simulink model "outerControllerTuning"  (R2018a)
settings: Solver=ode15s  StartTime=0.0  StopTime=t  RelTol=1e-3
values from neighbouring files (symbols this model uses):
  d = 2.4*10^-3    (= 0.0024)    [innerInit.m]    (also in outerInit.m)
  g = 9.81    [innerInit.m]    (also in outerInit.m)
  Ixx = 5.9*10^-3    (= 0.0059)    [innerInit.m]    (also in outerInit.m)
  Iyy = 5.9*10^-3    (= 0.0059)    [innerInit.m]    (also in outerInit.m)
  Izz = 1.16*10^-3    (= 0.00116)    [innerInit.m]    (also in outerInit.m)
  kr = 0.1    [innerInit.m]    (also in outerInit.m)
  kt = 0.1    [innerInit.m]    (also in outerInit.m)
  l = 0.255    [innerInit.m]    (also in outerInit.m)
  m = 0.5    [innerInit.m]    (also in outerInit.m)
  x0 = 1    [innerInit.m]    (also in outerInit.m = 2)
  x_coeff = A^-1*x_constr    [outerInit.m]
  xd = 0    [innerInit.m]    (also in outerInit.m)
  xdot0 = 0    [outerInit.m]
  y0 = 1    [innerInit.m]    (also in outerInit.m = 3)
  y_coeff = A^-1*y_constr    [outerInit.m]
  yd = 0    [innerInit.m]    (also in outerInit.m)
  ydot0 = 0    [outerInit.m]
  z0 = 0    [innerInit.m]    (also in outerInit.m = 4)
  z_coeff = A^-1*z_constr    [outerInit.m]
  zd = 10    [innerInit.m]    (also in outerInit.m = 0)
  zdot0 = 0    [outerInit.m]
libraries: simulink x4
settings Model: Creator=dinies33  LastModifiedBy=giuseppe

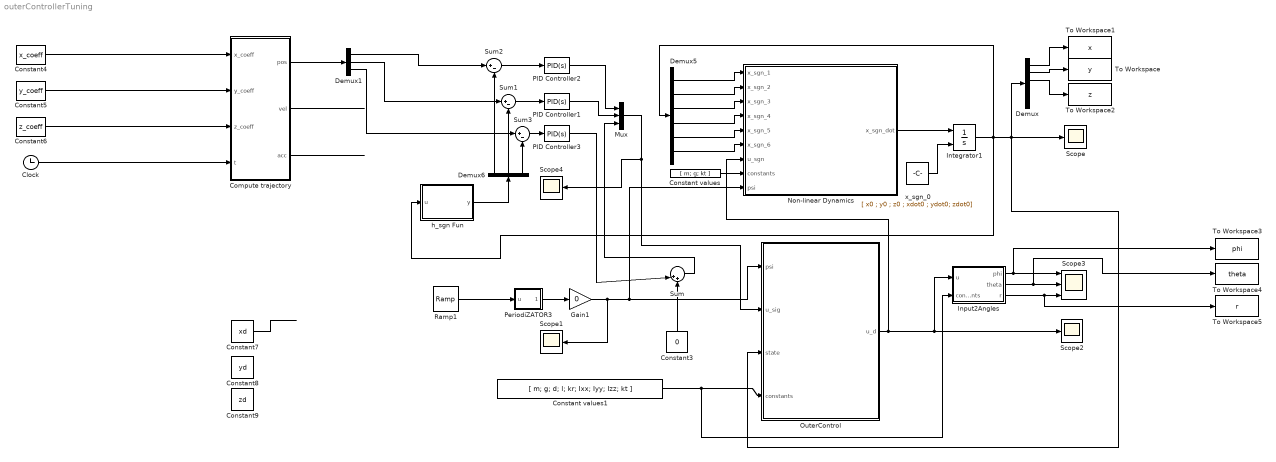
== system outerControllerTuning ==
  Clock : Clock
  Compute trajectory : MATLAB Function  TreatAsAtomicUnit=on
  Constant values : Constant  Value=[ m; g; kt ]
  Constant values1 : Constant  Value=[ m; g; d; l; kr; Ixx; Iyy; Izz; kt ]
  Constant3 : Constant  Value=0
  Constant4 : Constant  Value=x_coeff
  Constant5 : Constant  Value=y_coeff
  Constant6 : Constant  Value=z_coeff
  Constant7 : Constant  Value=xd
  Constant8 : Constant  Value=yd
  Constant9 : Constant  Value=zd
  Demux : Demux  Outputs=6
  Demux1 : Demux  Outputs=3
  Demux5 : Demux  Outputs=6
  Demux6 : Demux  Outputs=3
  Gain1 : Gain  Gain=0
  Input2Angles : MATLAB Function  TreatAsAtomicUnit=on
  Integrator1 : Integrator  InitialConditionSource=external
  Mux : Mux  Inputs=3
  Non-linear Dynamics : MATLAB Function  TreatAsAtomicUnit=on
  OuterControl : MATLAB Function  TreatAsAtomicUnit=on
  PID Controller1 : simulink/Continuous/PID Controller  Controller=PID  TimeDomain=Continuous-time  SampleTime=-1  IntegratorMethod=Forward Euler  FilterMethod=Forward Euler  Form=Parallel  UseFilter=on  ControllerParametersSource=internal  P=0.942155734377191  I=0.0299673249963071  D=20  N=509.539625142761  InitialConditionSource=internal  InitialConditionForIntegrator=0  InitialConditionForFilter=0  ExternalReset=none  LimitOutput=off  UpperSaturationLimit=inf  LowerSaturationLimit=-inf  LinearizeAsGain=on  AntiWindupMode=none  Kb=1  TrackingMode=off  Kt=1  PParamMin=[]  PParamMax=[]  IParamMin=[]  IParamMax=[]  DParamMin=[]  DParamMax=[]  NParamMin=[]  NParamMax=[]  KbParamMin=[]  KbParamMax=[]  KtParamMin=[]  KtParamMax=[]  POutMin=[]  POutMax=[]  IOutMin=[]  IOutMax=[]  DOutMin=[]  DOutMax=[]  NOutMin=[]  NOutMax=[]  KbOutMin=[]  KbOutMax=[]  KtOutMin=[]  KtOutMax=[]  IntegratorOutMin=[]  IntegratorOutMax=[]  FilterOutMin=[]  FilterOutMax=[]  SumOutMin=[]  SumOutMax=[]  SumI1OutMin=[]  SumI1OutMax=[]  SumI2OutMin=[]  SumI2OutMax=[]  SumI3OutMin=[]  SumI3OutMax=[]  SumDOutMin=[]  SumDOutMax=[]  SaturationOutMin=[]  SaturationOutMax=[]  IntegratorContinuousStateAttributes=''  IntegratorStateMustResolveToSignalObject=off  IntegratorRTWStateStorageClass=Auto  FilterContinuousStateAttributes=''  FilterStateMustResolveToSignalObject=off  FilterRTWStateStorageClass=Auto  DifferentiatorICPrevScaledInput=0  DifferentiatorOutMin=[]  DifferentiatorOutMax=[]  FilterDiffOutCoefMin=[]  FilterDiffOutCoefMax=[]  SumDenOutMin=[]  SumDenOutMax=[]  SumNumOutMin=[]  SumNumOutMax=[]  ReciprocalOutMin=[]  ReciprocalOutMax=[]  DivideOutMin=[]  DivideOutMax=[]  TunerSelectOption=Transfer Function Based (PID Tuner App)
  PID Controller2 : simulink/Continuous/PID Controller  Controller=PID  TimeDomain=Continuous-time  SampleTime=-1  IntegratorMethod=Forward Euler  FilterMethod=Forward Euler  Form=Parallel  UseFilter=on  ControllerParametersSource=internal  P=0.942155734377191  I=0.0299673249963071  D=20  N=509.539625142761  InitialConditionSource=internal  InitialConditionForIntegrator=0  InitialConditionForFilter=0  ExternalReset=none  LimitOutput=off  UpperSaturationLimit=inf  LowerSaturationLimit=-inf  LinearizeAsGain=on  AntiWindupMode=none  Kb=1  TrackingMode=off  Kt=1  PParamMin=[]  PParamMax=[]  IParamMin=[]  IParamMax=[]  DParamMin=[]  DParamMax=[]  NParamMin=[]  NParamMax=[]  KbParamMin=[]  KbParamMax=[]  KtParamMin=[]  KtParamMax=[]  POutMin=[]  POutMax=[]  IOutMin=[]  IOutMax=[]  DOutMin=[]  DOutMax=[]  NOutMin=[]  NOutMax=[]  KbOutMin=[]  KbOutMax=[]  KtOutMin=[]  KtOutMax=[]  IntegratorOutMin=[]  IntegratorOutMax=[]  FilterOutMin=[]  FilterOutMax=[]  SumOutMin=[]  SumOutMax=[]  SumI1OutMin=[]  SumI1OutMax=[]  SumI2OutMin=[]  SumI2OutMax=[]  SumI3OutMin=[]  SumI3OutMax=[]  SumDOutMin=[]  SumDOutMax=[]  SaturationOutMin=[]  SaturationOutMax=[]  IntegratorContinuousStateAttributes=''  IntegratorStateMustResolveToSignalObject=off  IntegratorRTWStateStorageClass=Auto  FilterContinuousStateAttributes=''  FilterStateMustResolveToSignalObject=off  FilterRTWStateStorageClass=Auto  DifferentiatorICPrevScaledInput=0  DifferentiatorOutMin=[]  DifferentiatorOutMax=[]  FilterDiffOutCoefMin=[]  FilterDiffOutCoefMax=[]  SumDenOutMin=[]  SumDenOutMax=[]  SumNumOutMin=[]  SumNumOutMax=[]  ReciprocalOutMin=[]  ReciprocalOutMax=[]  DivideOutMin=[]  DivideOutMax=[]  TunerSelectOption=Transfer Function Based (PID Tuner App)
  PID Controller3 : simulink/Continuous/PID Controller  Controller=PID  TimeDomain=Continuous-time  SampleTime=-1  IntegratorMethod=Forward Euler  FilterMethod=Forward Euler  Form=Parallel  UseFilter=on  ControllerParametersSource=internal  P=0.942155734377191  I=0.0299673249963071  D=30  N=509.539625142761  InitialConditionSource=internal  InitialConditionForIntegrator=0  InitialConditionForFilter=0  ExternalReset=none  LimitOutput=off  UpperSaturationLimit=inf  LowerSaturationLimit=-inf  LinearizeAsGain=on  AntiWindupMode=none  Kb=1  TrackingMode=off  Kt=1  PParamMin=[]  PParamMax=[]  IParamMin=[]  IParamMax=[]  DParamMin=[]  DParamMax=[]  NParamMin=[]  NParamMax=[]  KbParamMin=[]  KbParamMax=[]  KtParamMin=[]  KtParamMax=[]  POutMin=[]  POutMax=[]  IOutMin=[]  IOutMax=[]  DOutMin=[]  DOutMax=[]  NOutMin=[]  NOutMax=[]  KbOutMin=[]  KbOutMax=[]  KtOutMin=[]  KtOutMax=[]  IntegratorOutMin=[]  IntegratorOutMax=[]  FilterOutMin=[]  FilterOutMax=[]  SumOutMin=[]  SumOutMax=[]  SumI1OutMin=[]  SumI1OutMax=[]  SumI2OutMin=[]  SumI2OutMax=[]  SumI3OutMin=[]  SumI3OutMax=[]  SumDOutMin=[]  SumDOutMax=[]  SaturationOutMin=[]  SaturationOutMax=[]  IntegratorContinuousStateAttributes=''  IntegratorStateMustResolveToSignalObject=off  IntegratorRTWStateStorageClass=Auto  FilterContinuousStateAttributes=''  FilterStateMustResolveToSignalObject=off  FilterRTWStateStorageClass=Auto  DifferentiatorICPrevScaledInput=0  DifferentiatorOutMin=[]  DifferentiatorOutMax=[]  FilterDiffOutCoefMin=[]  FilterDiffOutCoefMax=[]  SumDenOutMin=[]  SumDenOutMax=[]  SumNumOutMin=[]  SumNumOutMax=[]  ReciprocalOutMin=[]  ReciprocalOutMax=[]  DivideOutMin=[]  DivideOutMax=[]  TunerSelectOption=Transfer Function Based (PID Tuner App)
  PeriodiZATOR3 : MATLAB Function  TreatAsAtomicUnit=on
  Ramp1 : simulink/Sources/Ramp  slope=0.3  start=0  InitialOutput=0
  Scope{,1..2,4} (4 alike) : Scope
  Scope3 : Scope  NumInputPorts=3
  Sum : Sum  Inputs=||++
  Sum1 : Sum  Inputs=|+-
  Sum2 : Sum  Inputs=|+-
  Sum3 : Sum  Inputs=|+-
  To Workspace : ToWorkspace  VariableName=y  SaveFormat=Timeseries  SampleTime=-1
  To Workspace1 : ToWorkspace  VariableName=x  SaveFormat=Timeseries  SampleTime=-1
  To Workspace2 : ToWorkspace  VariableName=z  SaveFormat=Timeseries  SampleTime=-1
  To Workspace3 : ToWorkspace  VariableName=phi  SaveFormat=Timeseries  SampleTime=-1
  To Workspace4 : ToWorkspace  VariableName=theta  SaveFormat=Timeseries  SampleTime=-1
  To Workspace5 : ToWorkspace  VariableName=r  SaveFormat=Timeseries  SampleTime=-1
  h_sgn Fun : MATLAB Function  TreatAsAtomicUnit=on
  x_sgn_0 : Constant  Value=[ x0 ; y0 ; z0 ; xdot0 ; ydot0; zdot0]
  wires:
  Constant values/1 -> Non-linear Dynamics/8(constants)
  Non-linear Dynamics/1(x_sgn_dot) -> Integrator1/1
  Integrator1/1 -> Demux5/1, OuterControl/3(state), Demux/1, Scope/1, h_sgn Fun/1(u)
  x_sgn_0/1 -> Integrator1/2
  Demux5/1 -> Non-linear Dynamics/1(x_sgn_1)
  Demux5/2 -> Non-linear Dynamics/2(x_sgn_2)
  Demux5/3 -> Non-linear Dynamics/3(x_sgn_3)
  Demux5/4 -> Non-linear Dynamics/4(x_sgn_4)
  Demux5/5 -> Non-linear Dynamics/5(x_sgn_5)
  Demux5/6 -> Non-linear Dynamics/6(x_sgn_6)
  Demux6/1 -> Sum2/2
  Demux6/2 -> Sum1/2
  h_sgn Fun/1(y) -> Demux6/1
  Sum3/1 -> PID Controller3/1
  Sum1/1 -> PID Controller1/1
  Sum2/1 -> PID Controller2/1
  Demux6/3 -> Sum3/2
  PID Controller2/1 -> Mux/1
  PID Controller1/1 -> Mux/2
  PID Controller3/1 -> Sum/1
  Sum/1 -> Mux/3
  Constant3/1 -> Sum/2
  Ramp1/1 -> PeriodiZATOR3/1(u)
  Constant values1/1 -> Input2Angles/2(constants), OuterControl/4(constants)
  Mux/1 -> Scope4/1, OuterControl/2(u_sig)
  OuterControl/1(u_d) -> Non-linear Dynamics/7(u_sgn), Input2Angles/1(u), Scope2/1
  Demux/1 -> To Workspace1/1
  Demux/2 -> To Workspace/1
  Demux/3 -> To Workspace2/1
  Input2Angles/1(phi) -> Scope3/1, To Workspace3/1
  Input2Angles/2(theta) -> Scope3/2, To Workspace4/1
  Input2Angles/3(r) -> To Workspace5/1, Scope3/3
  PeriodiZATOR3/1(angle) -> Gain1/1
  Compute trajectory/1(pos) -> Demux1/1
  Clock/1 -> Compute trajectory/4(t)
  Constant6/1 -> Compute trajectory/3(z_coeff)
  Constant5/1 -> Compute trajectory/2(y_coeff)
  Compute trajectory/2(vel) -> ?
  Compute trajectory/3(acc) -> ?
  Constant4/1 -> Compute trajectory/1(x_coeff)
  Gain1/1 -> Scope1/1, Non-linear Dynamics/9(psi), OuterControl/1(psi)
  Constant7/1 -> ?
  Demux1/1 -> Sum2/1
  Demux1/2 -> Sum1/1
  Demux1/3 -> Sum3/1

== matlab function outerControllerTuning/Input2Angles ==
  data: u input; phi output; constants input; theta output; r output
function [phi, theta, r] = fcn(u, constants)


m= constants(1,1);
d= constants(3,1);
kr= constants(5,1);

r = u(3)*d*m/kr;
phi = u(1)/u(3);
theta = u(2)/u(3);

== matlab function outerControllerTuning/h_sgn Fun ==
  data: u input; y output
function y = fcn(u)

h = [
    1 0 0 0 0 0;
    0 1 0 0 0 0;
    0 0 1 0 0 0;
    ];
    
y = h*u;

== matlab function outerControllerTuning/Compute trajectory ==
  data: x_coeff input; pos output; y_coeff input; z_coeff input; t input; vel output; acc output
function [pos, vel, acc]  = fcn(x_coeff, y_coeff, z_coeff, t)

x = x_coeff(1)*t^3+x_coeff(2)*t^2+x_coeff(3)*t+x_coeff(4);
y = y_coeff(1)*t^3+y_coeff(2)*t^2+y_coeff(3)*t+y_coeff(4);
z = z_coeff(1)*t^3+z_coeff(2)*t^2+z_coeff(3)*t+z_coeff(4);

x_dot = 3*x_coeff(1)*t^2 +2*x_coeff(2)*t + x_coeff(3);
y_dot = 3*y_coeff(1)*t^2 +2*y_coeff(2)*t + y_coeff(3);
z_dot = 3*z_coeff(1)*t^2 +2*z_coeff(2)*t + z_coeff(3);

x_ddot = 6*x_coeff(1)*t+2*x_coeff(2);
y_ddot = 6*y_coeff(1)*t+2*y_coeff(2);
z_ddot = 6*z_coeff(1)*t+2*z_coeff(2);

u = zeros(3,1);

pos = [x, y, z]';
vel = [x_dot, y_dot, z_dot]';
acc = [x_ddot, y_ddot, z_ddot]';

== matlab function outerControllerTuning/Non-linear Dynamics ==
  data: x_sgn_1 input; x_sgn_dot output; x_sgn_2 input; x_sgn_3 input; x_sgn_4 input; x_sgn_5 input; x_sgn_6 input; u_sgn input; constants input; psi input
function x_sgn_dot = fcn(x_sgn_1,x_sgn_2,x_sgn_3,x_sgn_4,x_sgn_5,x_sgn_6,u_sgn,constants, psi)
 
m= constants(1,1);
g= constants(2,1);
kt = constants(3,1);
 
% x_sgn = [x_sgn_1;
%         x_sgn_2;
%         x_sgn_3;
%         x_sgn_4;
%         x_sgn_5;
%         x_sgn_6];
    
% A = zeros(6);
% A(1:3,4:6) = eye(3);
% A(4:6,4:6) = -kt*m*eye(3);
% 
% G= zeros(6,3);
% G(4:6,:) = eye(3);

f = [x_sgn_4; 
     x_sgn_5;
     x_sgn_6;
     cos(psi)*u_sgn(2) + sin(psi)*u_sgn(1) - kt/m*x_sgn_4;
     sin(psi)*u_sgn(2) - cos(psi)*u_sgn(1) - kt/m*x_sgn_5;
     u_sgn(3) - kt/m*x_sgn_6 - g];


% x_sgn_dot = A*x_sgn + G*u_sgn_sgn + [ 0 0 0 0 0 -g]' ;
x_sgn_dot = f;

== matlab function outerControllerTuning/OuterControl ==
  data: psi input; u_d output; u_sig input; state input; constants input
function u_d = fcn(psi, u_sig, state, constants)

m= constants(1,1);
d= constants(3,1);
kr= constants(5,1);
kt = constants(9,1); 

u1_sig_sig = u_sig(1);
u2_sig_sig = u_sig(2);
u3_sig = u_sig(3);

R = [sin(psi), cos(psi);
    -cos(psi), sin(psi)];

u_sig_sig = [(u1_sig_sig) (u2_sig_sig)]';
% kt/m*state(4)
u12 = R'*u_sig_sig;

u_d = [0 0 0]';
u_d(1) = u12(1);
u_d(2)= u12(2);
u_d(3) = u3_sig+9.81; % + kt/m*state(6);

== matlab function outerControllerTuning/PeriodiZATOR3 ==
  data: u input; angle output
function angle = fcn(u)

y = sin(u);
x = cos(u);

% angle = mod(u, 2*pi);
angle = atan2(y,x);
